simulink model "demo"  (R2020a)
settings: Solver=VariableStepAuto  StartTime=0.0  StopTime=5  RelTol=1e-3
values from neighbouring files (symbols this model uses):
  header = [src,dst,message_type, data_type, priority, option,flag,param,subparam]    [api.m]
libraries: sldrtlib x1, xpcutilitieslib x1, xpcrtudplib x1
settings Model: PacingRate=0.001000  Creator=Chuanyu Xue  LastModifiedBy=Chuanyu Xue

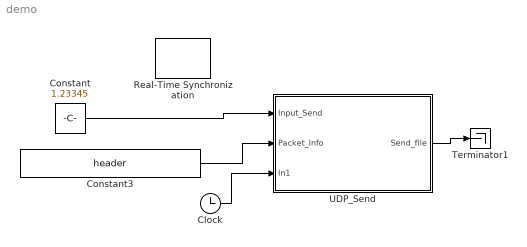
== system demo ==
  Clock : Clock
  Constant : Constant  Value=1.23345  SampleTime=1
  Constant3 : Constant  Value=header  SampleTime=1
  Real-Time Synchronization : sldrtlib/Real-Time Synchronization  SampleTime=10  MaxMissedTicks=10  ShowMissedTicks=off  YieldWhenWaiting=off
  Terminator1 : Terminator
  UDP_Send : Subsystem
  wires:
  UDP_Send/1(Send_file) -> Terminator1/1
  Constant3/1 -> UDP_Send/2(Packet_Info)
  Constant/1 -> UDP_Send/1(Input_Send)
  Clock/1 -> UDP_Send/3(In1)

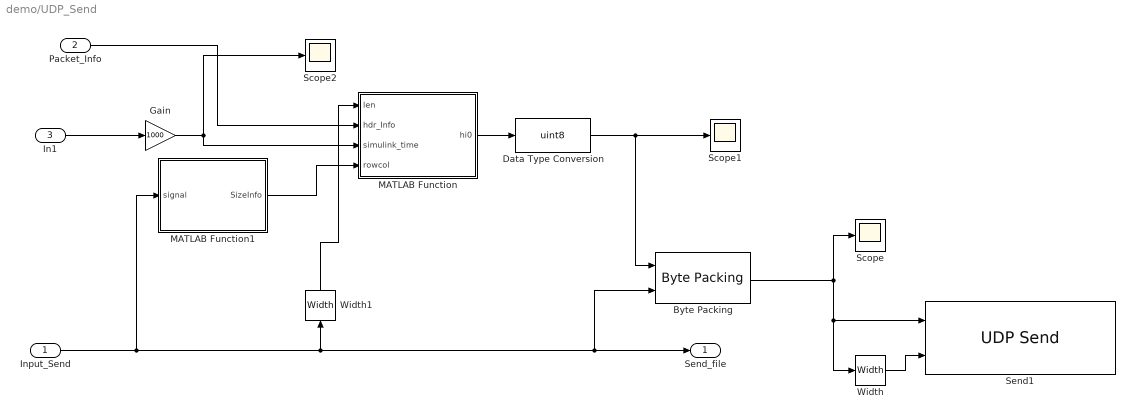
== system demo/UDP_Send ==
  Input_Send : Inport
  Packet_Info : Inport  Port=2
  In1 : Inport  Port=3
  "Byte Packing " : xpcutilitieslib/Byte Packing   MaskPackedDataType=uint8  MaskUnpackedDataTypes={'uint8','double'}  MaskAlignment=1
  Data Type Conversion : DataTypeConversion  OutDataTypeStr=uint8
  Gain : Gain  Gain=1000
  MATLAB Function : MATLAB Function  TreatAsAtomicUnit=on
  MATLAB Function1 : MATLAB Function  TreatAsAtomicUnit=on
  Scope : Scope
  Scope1 : Scope
  Scope2 : Scope
  Send1 : xpcrtudplib/UDP Send  ipAddressVal=Use host-target connection  localPort=l_port  toAddress=remote_ip  toPort=r_port  sampleTime=1
      settings: SourceProductBaseCode=XP
  Width : Width
  Width1 : Width
  Send_file : Outport
  wires:
  Width1/1 -> MATLAB Function/1(len)
  Input_Send/1 -> "Byte Packing "/2, Send_file/1, Width1/1, MATLAB Function1/1(signal)
  "Byte Packing "/1 -> Scope/1, Width/1, Send1/1
  Width/1 -> Send1/2
  MATLAB Function/1(hi0) -> Data Type Conversion/1
  Data Type Conversion/1 -> Scope1/1, "Byte Packing "/1
  Packet_Info/1 -> MATLAB Function/2(hdr_Info)
  MATLAB Function1/1(SizeInfo) -> MATLAB Function/4(rowcol)
  Gain/1 -> Scope2/1, MATLAB Function/3(simulink_time)
  In1/1 -> Gain/1

== matlab function demo/UDP_Send/MATLAB Function ==
  data: hi0 output; len input; hdr_Info input; simulink_time input; rowcol input
function hi0 =headerInfo(len, hdr_Info, simulink_time, rowcol)
% 4 bit
src=hdr_Info(1);
% 4 bit
dst=hdr_Info(2);
% 4 bit
message_type = hdr_Info(3);
% 8 bit
data_type = hdr_Info(4);
% 4 bit
priority = hdr_Info(5);
mix = bitshift(message_type, 12) + bitshift(data_type, 4) + priority;
% 32 bit
%physical_time =uint32(2345678910);
physical_time = uint32(posixtime(datetime('now')));
% 32 bit
simulink_time = uint32(simulink_time);
% 8 bit
row=rowcol(1); 
% 8 bit
col=rowcol(2);
% 16 bit
length = len;
% 16 bit
option = hdr_Info(6);
% 16 bit
flag = hdr_Info(7);
% 16 bit
param = hdr_Info(8);
% 16 bit
subparam = hdr_Info(9);


% make everything 8 bit:
o1 = src;
o2 = dst;
o3 = bitshift(mix, -8);
o4 = bitand(mix, 256);

o5 = bitand(bitshift(physical_time, -24), 256);
o6 = bitand(bitshift(physical_time, -16), 256);
o7 = bitand(bitshift(physical_time, -8), 256);
o8 = bitand(physical_time, 256);


o9 = bitand(bitshift(simulink_time, -24), 256);
o10 = bitand(bitshift(simulink_time, -16), 256);
o11 = bitand(bitshift(simulink_time, -8), 256);
o12 = bitand(simulink_time, 256);

o13 = row;
o14 = col;
o15 = bitshift(length, -8);
o16 = bitand(length, 256);

o17 = bitshift(option, -8);
o18 = bitand(option, 256);
o19 = bitshift(flag, -8);
o20 = bitand(flag, 256);

o21 = bitshift(param, -8);
o22 = bitand(param, 256);
o23 = bitshift(subparam, -8);
o24 = bitand(subparam, 256);

% 8 bit headers 
hi0=[o1, o2, o3, o4, o5, o6, o7, o8, o9, o10, o11, o12, o13, o14, o15, o16, o17, o18, o19, o20, o21, o22, o23, o24];
% hi0 = [1,2,3,4,5,6];
% hi=uint8(hi);

== matlab function demo/UDP_Send/MATLAB Function1 ==
  data: SizeInfo output; signal input
function SizeInfo=size_Info(signal)

info=size(signal);

SizeInfo=[info(1), info(2)];
